simulink model "aero"  (R2020b)
settings: Solver=VariableStepAuto  StartTime=0.0  StopTime=10.0  RelTol=1e-3
undefined symbols (not defined in the file or in its folder): par
settings Model: Creator=Tjeu  LastModifiedBy=Tjeu
settings DebuggingCC: UnconnectedInputMsg=none  UnconnectedOutputMsg=none  UnconnectedLineMsg=none  SFMachineParentedDataDiag=error

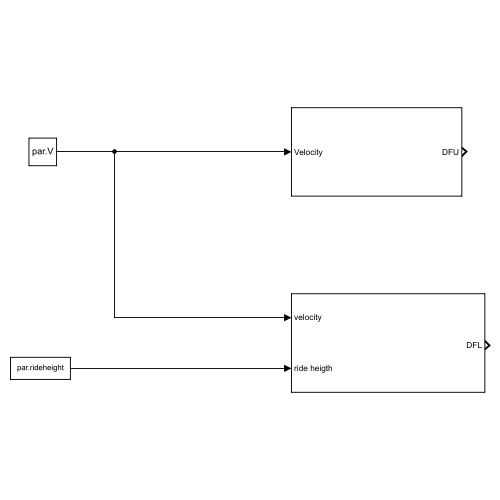
[thumbnail: Simulink's stored preview of the top-level diagram]
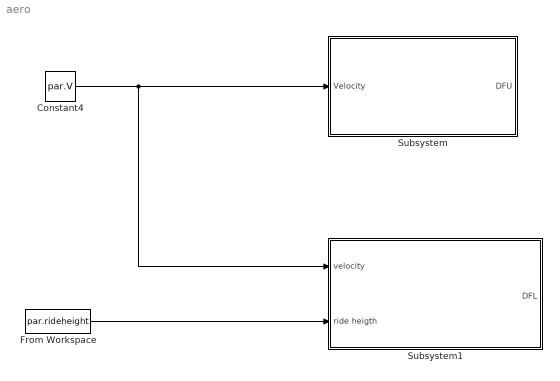
== system aero ==
  Constant4 : Constant  Value=par.V
  From Workspace : FromWorkspace  VariableName=par.rideheight
  Subsystem : Subsystem
  Subsystem1 : Subsystem
  wires:
  Constant4/1 -> Subsystem1/1(velocity), Subsystem/1(Velocity)
  From Workspace/1 -> Subsystem1/2(ride heigth)

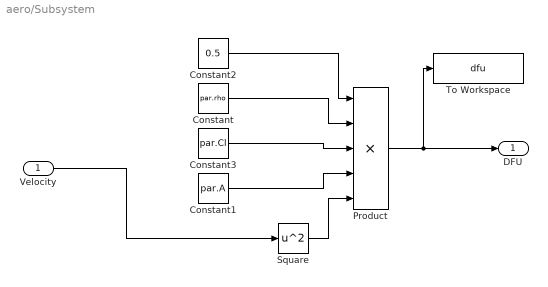
== system aero/Subsystem ==
  Velocity : Inport
  Constant : Constant  Value=par.rho
  Constant1 : Constant  Value=par.A
  Constant2 : Constant  Value=0.5
  Constant3 : Constant  Value=par.Cl
  Product : Product  Inputs=5
  Square : Math  Operator=square  SaturateOnIntegerOverflow=on
  To Workspace : ToWorkspace  VariableName=dfu  SaveFormat=Timeseries  SampleTime=-1
  DFU : Outport
  wires:
  Constant2/1 -> Product/1
  Constant/1 -> Product/2
  Constant1/1 -> Product/4
  Constant3/1 -> Product/3
  Square/1 -> Product/5
  Product/1 -> To Workspace/1, DFU/1
  Velocity/1 -> Square/1

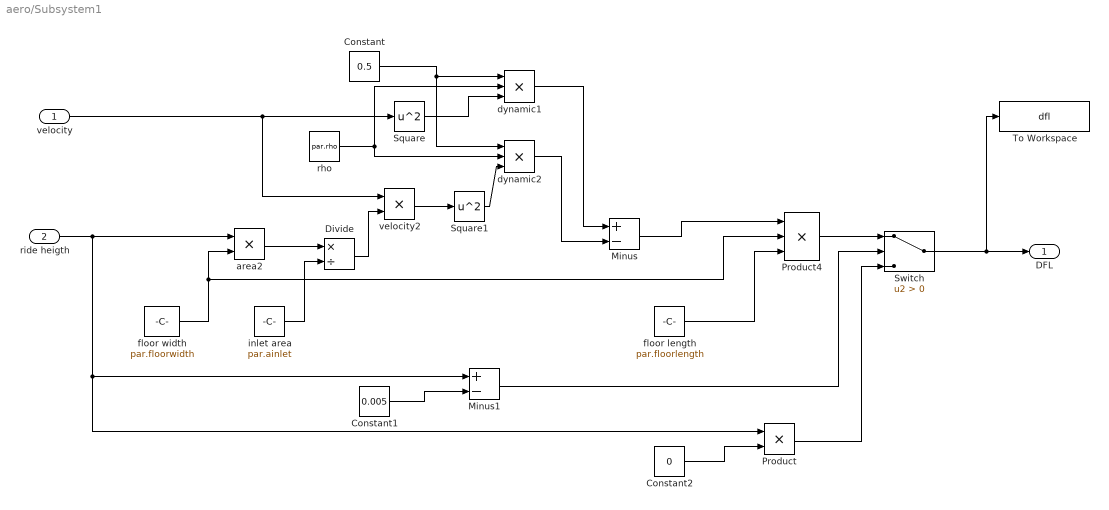
== system aero/Subsystem1 ==
  velocity : Inport
  ride heigth : Inport  Port=2
  Constant : Constant  Value=0.5
  Constant1 : Constant  Value=0.005
  Constant2 : Constant  Value=0
  Divide : Product  Inputs=*/
  Minus : Sum  Inputs=+-
  Minus1 : Sum  Inputs=+-
  Product : Product
  Product4 : Product  Inputs=3
  Square : Math  Operator=square  SaturateOnIntegerOverflow=on
  Square1 : Math  Operator=square  SaturateOnIntegerOverflow=on
  Switch : Switch  Criteria=u2 > Threshold
  To Workspace : ToWorkspace  VariableName=dfl  SaveFormat=Timeseries  SampleTime=-1
  area2 : Product
  dynamic1 : Product  Inputs=3
  dynamic2 : Product  Inputs=3
  floor length : Constant  Value=par.floorlength
  floor width : Constant  Value=par.floorwidth
  inlet area : Constant  Value=par.ainlet
  rho : Constant  Value=par.rho
  velocity2 : Product
  DFL : Outport
  wires:
  Square1/1 -> dynamic2/3
  dynamic1/1 -> Minus/1
  Divide/1 -> velocity2/2
  area2/1 -> Divide/1
  rho/1 -> dynamic1/2, dynamic2/2
  floor width/1 -> Product4/2, area2/2
  velocity/1 -> Square/1, velocity2/1
  dynamic2/1 -> Minus/2
  floor length/1 -> Product4/3
  Minus/1 -> Product4/1
  Square/1 -> dynamic1/3
  Constant/1 -> dynamic2/1, dynamic1/1
  ride heigth/1 -> Product/1, Minus1/1, area2/1
  velocity2/1 -> Square1/1
  inlet area/1 -> Divide/2
  Product4/1 -> Switch/1
  Constant1/1 -> Minus1/2
  Minus1/1 -> Switch/2
  Constant2/1 -> Product/2
  Product/1 -> Switch/3
  Switch/1 -> To Workspace/1, DFL/1
